simulink model "week06_basebot_test"  (R2026a)
settings: Solver=ode45  StopTime=3  MaxStep=min([wheels.Ts])/10  RelTol=1e-6  AbsTol=1e-9
model workspace (MAT data in the model file):
  referenceSpeed = [0.1 0.1]
  stepTime = 0.2
  wheels(1).L = 0.00768482381376
  wheels(1).R = 6.41139804096
  wheels(1).Kt = 0.0102935612741
  wheels(1).Kb = 0.0102935612741
  wheels(1).J = 5.4618603579e-06
  wheels(1).D = 6.52401278375e-07
  wheels(1).gear = 9.68
  wheels(1).wheelRadius = 0.03
  wheels(1).Kp = 2.03180408642
  wheels(1).Ts = 0.001
  wheels(1).voltageLimit = 9
  wheels(2).L = 0.00332761119549
  wheels(2).R = 2.86396181384
  wheels(2).Kt = 0.00798363352314
  wheels(2).Kb = 0.00798363352314
  wheels(2).J = 5.4618603579e-06
  wheels(2).D = 3.3790070145e-06
  wheels(2).gear = 9.68
  wheels(2).wheelRadius = 0.03
  wheels(2).Kp = 0.766619928019
  wheels(2).Ts = 0.001
  wheels(2).voltageLimit = 9
values from neighbouring files (symbols this model uses):
  wheels =     [basebot_test_results.mat]    (also in robot_model_defaults.m = tuned.motorParameters; run_basebot_test.m = repmat(struct('L',0,'R',0,'Kt',0,'Kb',0,'J',0,'D',0,      'g)
settings Model: Creator=michaeljohansen  LastModifiedBy=michaeljohansen

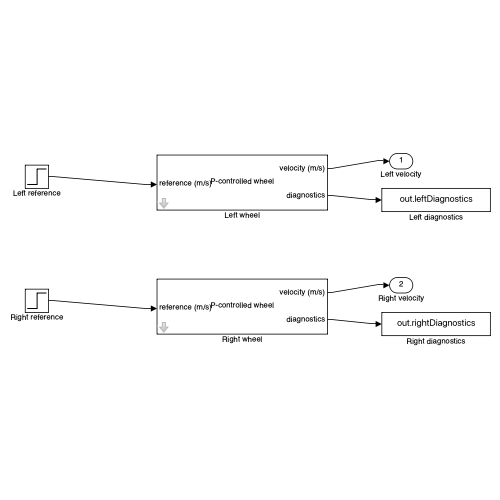
[thumbnail: Simulink's stored preview of the top-level diagram]
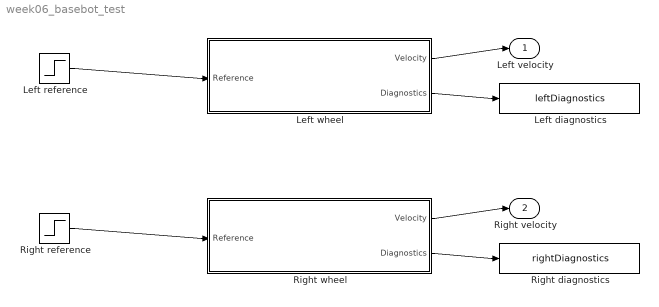
== system week06_basebot_test ==
  Left diagnostics : ToWorkspace  VariableName=leftDiagnostics  SaveFormat=Timeseries  SampleTime=-1
  Left reference : Step  Time=stepTime  FinalValue=referenceSpeed(1)  SampleTime=0
  Left wheel : Subsystem  mask{L=wheels(1).L, R=wheels(1).R, Kt=wheels(1).Kt, Kb=wheels(1).Kb, J=wheels(1).J, D=wheels(1).D, gear=wheels(1).gear, wheelRadius=wheels(1).wheelRadius, Kp=wheels(1).Kp, Ts=wheels(1).Ts, voltageLimit=wheels(1).voltageLimit}
      mask Display: disp('P-controlled wheel'); port_label('input',1,'reference (m/s)'); port_label('output',1,'velocity (m/s)'); port_label('output',2,'diagnostics');
  Right diagnostics : ToWorkspace  VariableName=rightDiagnostics  SaveFormat=Timeseries  SampleTime=-1
  Right reference : Step  Time=stepTime  FinalValue=referenceSpeed(2)  SampleTime=0
  Right wheel : Subsystem  mask{L=wheels(2).L, R=wheels(2).R, Kt=wheels(2).Kt, Kb=wheels(2).Kb, J=wheels(2).J, D=wheels(2).D, gear=wheels(2).gear, wheelRadius=wheels(2).wheelRadius, Kp=wheels(2).Kp, Ts=wheels(2).Ts, voltageLimit=wheels(2).voltageLimit}
      mask Display: disp('P-controlled wheel'); port_label('input',1,'reference (m/s)'); port_label('output',1,'velocity (m/s)'); port_label('output',2,'diagnostics');
  Left velocity : Outport
  Right velocity : Outport  Port=2
  wires:
  Left reference/1 -> Left wheel/1(Reference)
  Left wheel/1(Velocity) -> Left velocity/1
  Left wheel/2(Diagnostics) -> Left diagnostics/1
  Right reference/1 -> Right wheel/1(Reference)
  Right wheel/1(Velocity) -> Right velocity/1
  Right wheel/2(Diagnostics) -> Right diagnostics/1

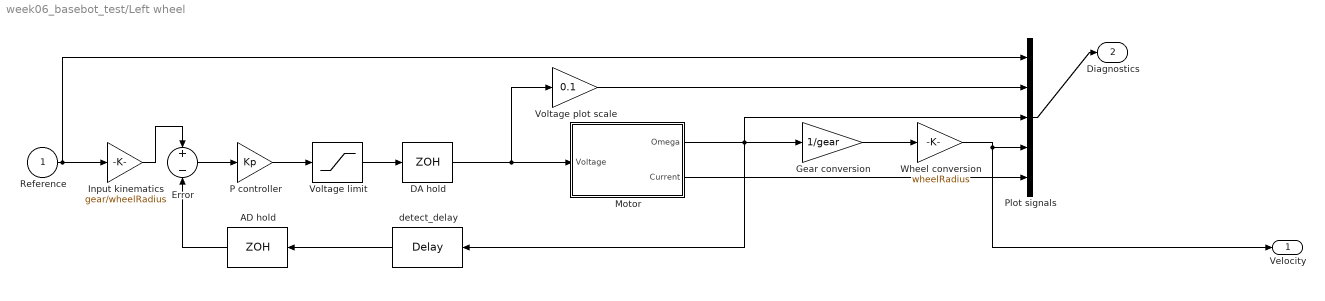
== system week06_basebot_test/Left wheel ==
  Reference : Inport
  AD hold : ZeroOrderHold  SampleTime=Ts
  DA hold : ZeroOrderHold  SampleTime=Ts
  Error : Sum  Inputs=+-
  Gear conversion : Gain  Gain=1/gear
  Input kinematics : Gain  Gain=gear/wheelRadius
  Motor : Subsystem
  P controller : Gain  Gain=Kp
  Plot signals : Mux  Inputs=5
  Voltage limit : Saturate  UpperLimit=voltageLimit  LowerLimit=-voltageLimit
  Voltage plot scale : Gain  Gain=0.1
  Wheel conversion : Gain  Gain=wheelRadius
  detect_delay : TransportDelay  DelayTime=Ts
  Velocity : Outport
  Diagnostics : Outport  Port=2
  wires:
  P controller/1 -> Voltage limit/1
  Error/1 -> P controller/1
  Voltage plot scale/1 -> Plot signals/2
  DA hold/1 -> Voltage plot scale/1, Motor/1(Voltage)
  AD hold/1 -> Error/2
  Gear conversion/1 -> Wheel conversion/1
  Input kinematics/1 -> Error/1
  detect_delay/1 -> AD hold/1
  Voltage limit/1 -> DA hold/1
  Motor/1(Omega) -> Plot signals/3, Gear conversion/1, detect_delay/1
  Wheel conversion/1 -> Plot signals/4, Velocity/1
  Motor/2(Current) -> Plot signals/5
  Reference/1 -> Input kinematics/1, Plot signals/1
  Plot signals/1 -> Diagnostics/1

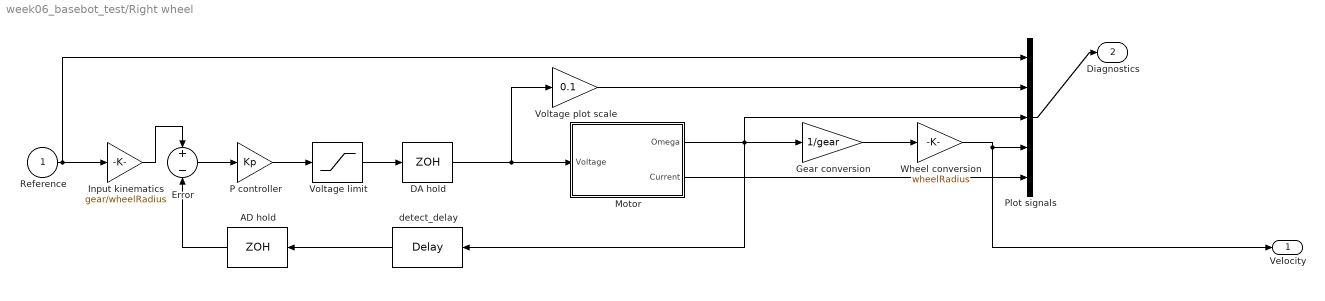
== system week06_basebot_test/Right wheel ==
  Reference : Inport
  AD hold : ZeroOrderHold  SampleTime=Ts
  DA hold : ZeroOrderHold  SampleTime=Ts
  Error : Sum  Inputs=+-
  Gear conversion : Gain  Gain=1/gear
  Input kinematics : Gain  Gain=gear/wheelRadius
  Motor : Subsystem
  P controller : Gain  Gain=Kp
  Plot signals : Mux  Inputs=5
  Voltage limit : Saturate  UpperLimit=voltageLimit  LowerLimit=-voltageLimit
  Voltage plot scale : Gain  Gain=0.1
  Wheel conversion : Gain  Gain=wheelRadius
  detect_delay : TransportDelay  DelayTime=Ts
  Velocity : Outport
  Diagnostics : Outport  Port=2
  wires:
  P controller/1 -> Voltage limit/1
  Error/1 -> P controller/1
  Voltage plot scale/1 -> Plot signals/2
  DA hold/1 -> Voltage plot scale/1, Motor/1(Voltage)
  AD hold/1 -> Error/2
  Gear conversion/1 -> Wheel conversion/1
  Input kinematics/1 -> Error/1
  detect_delay/1 -> AD hold/1
  Voltage limit/1 -> DA hold/1
  Motor/1(Omega) -> Plot signals/3, Gear conversion/1, detect_delay/1
  Wheel conversion/1 -> Plot signals/4, Velocity/1
  Motor/2(Current) -> Plot signals/5
  Reference/1 -> Input kinematics/1, Plot signals/1
  Plot signals/1 -> Diagnostics/1

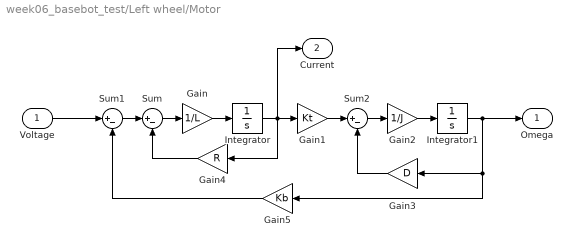
== system week06_basebot_test/Left wheel/Motor ==
  Voltage : Inport
  Gain : Gain  Gain=1/L
  Gain1 : Gain  Gain=Kt
  Gain2 : Gain  Gain=1/J
  Gain3 : Gain  Gain=D
  Gain4 : Gain  Gain=R
  Gain5 : Gain  Gain=Kb
  Integrator : Integrator
  Integrator1 : Integrator
  Sum : Sum  Inputs=|+-
  Sum1 : Sum  Inputs=|+-
  Sum2 : Sum  Inputs=|+-
  Omega : Outport
  Current : Outport  Port=2
  wires:
  Gain5/1 -> Sum1/2
  Gain3/1 -> Sum2/2
  Integrator1/1 -> Omega/1, Gain5/1, Gain3/1
  Gain2/1 -> Integrator1/1
  Sum2/1 -> Gain2/1
  Gain1/1 -> Sum2/1
  Gain4/1 -> Sum/2
  Integrator/1 -> Current/1, Gain4/1, Gain1/1
  Gain/1 -> Integrator/1
  Sum/1 -> Gain/1
  Sum1/1 -> Sum/1
  Voltage/1 -> Sum1/1

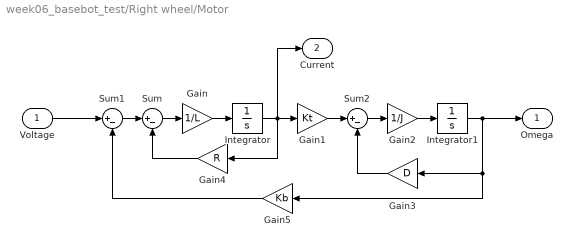
== system week06_basebot_test/Right wheel/Motor ==
  Voltage : Inport
  Gain : Gain  Gain=1/L
  Gain1 : Gain  Gain=Kt
  Gain2 : Gain  Gain=1/J
  Gain3 : Gain  Gain=D
  Gain4 : Gain  Gain=R
  Gain5 : Gain  Gain=Kb
  Integrator : Integrator
  Integrator1 : Integrator
  Sum : Sum  Inputs=|+-
  Sum1 : Sum  Inputs=|+-
  Sum2 : Sum  Inputs=|+-
  Omega : Outport
  Current : Outport  Port=2
  wires:
  Gain5/1 -> Sum1/2
  Gain3/1 -> Sum2/2
  Integrator1/1 -> Omega/1, Gain5/1, Gain3/1
  Gain2/1 -> Integrator1/1
  Sum2/1 -> Gain2/1
  Gain1/1 -> Sum2/1
  Gain4/1 -> Sum/2
  Integrator/1 -> Current/1, Gain4/1, Gain1/1
  Gain/1 -> Integrator/1
  Sum/1 -> Gain/1
  Sum1/1 -> Sum/1
  Voltage/1 -> Sum1/1
